simulink model "systeme_2018a"  (R2018a)
settings: Solver=VariableStepAuto  StartTime=0.0  StopTime=10  RelTol=1e-3
libraries: simulink x1
settings Model: Creator=etell  LastModifiedBy=Ethan Ellison
settings DataIOCC: ReturnWorkspaceOutputs=on
settings SFSimCC: SimUseLocalCustomCode=on
settings RTWCC: RTWUseLocalCustomCode=on

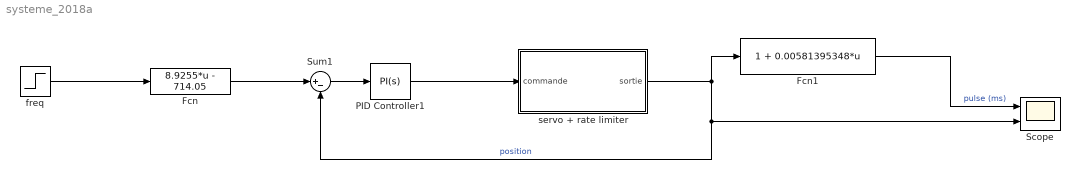
== system systeme_2018a ==
  Fcn : Fcn  Expr=8.9255*u - 714.05
  Fcn1 : Fcn  Expr=1 + 0.00581395348*u
  PID Controller1 : simulink/Continuous/PID Controller  Controller=PI  Form=Parallel  TimeDomain=Continuous-time  SampleTime=-1  IntegratorMethod=Forward Euler  FilterMethod=Forward Euler  ControllerParametersSource=internal  P=0.5  I=10  D=0  UseFilter=on  N=100  TunerSelectOption=Transfer Function Based (PID Tuner App)  InitialConditionSource=internal  InitialConditionForIntegrator=0  InitialConditionForFilter=0  DifferentiatorICPrevScaledInput=0  ExternalReset=none  TrackingMode=off  Kt=1  LimitOutput=on  UpperSaturationLimit=172  LowerSaturationLimit=0  LinearizeAsGain=on  AntiWindupMode=none  Kb=1  POutMin=[]  POutMax=[]  IOutMin=[]  IOutMax=[]  DOutMin=[]  DOutMax=[]  NOutMin=[]  NOutMax=[]  SumOutMin=[]  SumOutMax=[]  SaturationOutMin=[]  SaturationOutMax=[]  PParamMin=[]  PParamMax=[]  IParamMin=[]  IParamMax=[]  DParamMin=[]  DParamMax=[]  NParamMin=[]  NParamMax=[]  KbParamMin=[]  KbParamMax=[]  KtParamMin=[]  KtParamMax=[]  KbOutMin=[]  KbOutMax=[]  KtOutMin=[]  KtOutMax=[]  IntegratorOutMin=[]  IntegratorOutMax=[]  FilterOutMin=[]  FilterOutMax=[]  SumI1OutMin=[]  SumI1OutMax=[]  SumI2OutMin=[]  SumI2OutMax=[]  SumI3OutMin=[]  SumI3OutMax=[]  SumDOutMin=[]  SumDOutMax=[]  DifferentiatorOutMin=[]  DifferentiatorOutMax=[]  FilterDiffOutCoefMin=[]  FilterDiffOutCoefMax=[]  ReciprocalOutMin=[]  ReciprocalOutMax=[]  SumDenOutMin=[]  SumDenOutMax=[]  SumNumOutMin=[]  SumNumOutMax=[]  DivideOutMin=[]  DivideOutMax=[]  IntegratorContinuousStateAttributes=''  IntegratorStateMustResolveToSignalObject=off  IntegratorRTWStateStorageClass=Auto  FilterContinuousStateAttributes=''  FilterStateMustResolveToSignalObject=off  FilterRTWStateStorageClass=Auto
  Scope : Scope  NumInputPorts=2
  Sum1 : Sum  Inputs=|+-
  "freq " : Step  Time=3  Before=80  After=120  SampleTime=0
  "servo + rate limiter " : Subsystem
  wires:
  "servo + rate limiter "/1("sortie ") -> Fcn1/1, Scope/2, Sum1/2  "position"
  PID Controller1/1 -> "servo + rate limiter "/1("commande ")
  Sum1/1 -> PID Controller1/1
  Fcn/1 -> Sum1/1
  "freq "/1 -> Fcn/1
  Fcn1/1 -> Scope/1  "pulse (ms)"

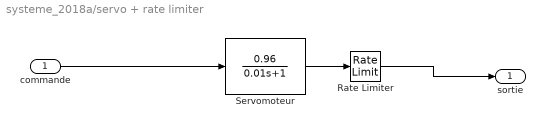
== system systeme_2018a/servo + rate limiter  ==
  "commande " : Inport
  Rate Limiter : RateLimiter  RisingSlewLimit=238.6  FallingSlewLimit=-238.6  SampleTimeMode=inherited
  "Servomoteur " : TransferFcn  Numerator=[0.96]  Denominator=[0.01 1]
  "sortie " : Outport
  wires:
  "Servomoteur "/1 -> Rate Limiter/1
  Rate Limiter/1 -> "sortie "/1
  "commande "/1 -> "Servomoteur "/1
